simulink model "generic_Truck_And_Trailer"  (R2025a)
settings: Solver=VariableStepAuto  StartTime=0.0  StopTime=350  FixedStep=0.01  MaxStep=0.001  RelTol=1e-3  EnableMultiTasking=on
libraries: TruckMaker4SL x250, simulink x1
(part 3 of 11)

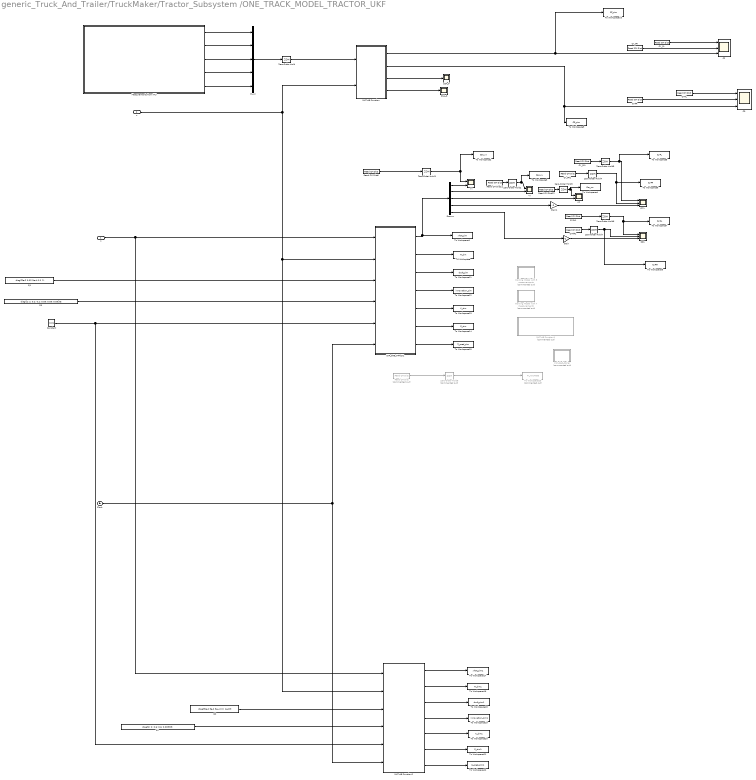
== system generic_Truck_And_Trailer/TruckMaker/Tractor_Subsystem /ONE_TRACK_MODEL_TRACTOR_UKF ==
  z : Inport
  u : Inport  Port=2
  "CF " : Scope  NumInputPorts=3
      settings: ActiveDisplayYMinimum=-12.263034323337607  ActiveDisplayYMaximum=-4.9489164501428942  DataLoggingVariableName=ScopeData23
  CF 1 : Scope  NumInputPorts=3
      settings: ActiveDisplayYMinimum=-10.797860186662938  ActiveDisplayYMaximum=-3.0037046797887497  DataLoggingVariableName=ScopeData30
  CR : Scope  NumInputPorts=3
      settings: ActiveDisplayYMinimum=-11.701585356235972  ActiveDisplayYMaximum=4.5045535239425494  DataLoggingVariableName=ScopeData24
  CR1 : Scope  NumInputPorts=3
      settings: ActiveDisplayYMinimum=-13.474282112558932  ActiveDisplayYMaximum=-8.0648262356989679  DataLoggingVariableName=ScopeData31
  CYRL : TruckMaker4SL/Read CM Dict  xname=CyRL  xsync=off  xstime=Continuous
      settings: SourceProductName=TruckMaker4SL
  CYRL1 : TruckMaker4SL/Read CM Dict  xname=CyRL  xsync=off  xstime=Continuous
      settings: SourceProductName=TruckMaker4SL
  CYRR : TruckMaker4SL/Read CM Dict  xname=CyRR  xsync=off  xstime=Continuous
      settings: SourceProductName=TruckMaker4SL
  CYRR1 : TruckMaker4SL/Read CM Dict  xname=CyRR  xsync=off  xstime=Continuous
      settings: SourceProductName=TruckMaker4SL
  CY_FL : TruckMaker4SL/Read CM Dict  xname=CyFL  xsync=off  xstime=Continuous
      settings: SourceProductName=TruckMaker4SL
  CY_FL1 : TruckMaker4SL/Read CM Dict  xname=CyFL  xsync=off  xstime=Continuous
      settings: SourceProductName=TruckMaker4SL
  CY_FR : TruckMaker4SL/Read CM Dict  xname=CyFR  xsync=off  xstime=Continuous
      settings: SourceProductName=TruckMaker4SL
  CY_FR1 : TruckMaker4SL/Read CM Dict  xname=CyFR  xsync=off  xstime=Continuous
      settings: SourceProductName=TruckMaker4SL
  Clock : Clock
  Constant : Constant  Value=0.01
  Demux : Demux  Outputs=5
  Gain : Gain  Gain=-1
  Gain1 : Gain  Gain=-1
  "Included_trailer " : MATLAB Function  Commented=on  TreatAsAtomicUnit=on
  MATLAB Function : MATLAB Function  TreatAsAtomicUnit=on
  MATLAB Function1 : MATLAB Function  Commented=on  TreatAsAtomicUnit=on
  MATLAB Function2 : MATLAB Function  TreatAsAtomicUnit=on  SystemSampleTime=0.01
  Measurements from IMU : Subsystem  Description=Measurements from IMU Mounted in Vhcl position (3.6; 0.0;1.0)
  Mux2 : Mux  Inputs=5
  Q1 : Constant  Value="diag([2e-2 0.02 3e-4 0 0  ]);"
  Q2 : Constant  Value="diag([5e-2 5e-2 3e-4 0 0  1e-3]);"
  R1 : Constant  Value=diag([2; 2; 0.6; 0.6; 0.005])/3;
  R3 : Constant  Value=diag([2; 2; 0.2; 0.2; 0.05; 0.05; 0.05])/3;
  Read CM Dict : TruckMaker4SL/Read CM Dict  Commented=on  xname=Tr.YawVel  xsync=off  xstime=Continuous
      settings: SourceProductName=TruckMaker4SL
  Read CM Dict11 : TruckMaker4SL/Read CM Dict  xname=Car.vy  xsync=off  xstime=Continuous
      settings: SourceProductName=TruckMaker4SL
  Read CM Dict12 : TruckMaker4SL/Read CM Dict  xname=Car.YawRate  xsync=off  xstime=Continuous
      settings: SourceProductName=TruckMaker4SL
  Read CM Dict6 : TruckMaker4SL/Read CM Dict  xname=Car.vx  xsync=off  xstime=Continuous
      settings: SourceProductName=TruckMaker4SL
  SSA_F : Scope
      settings: ActiveDisplayYMinimum=-0.046315426334515186  ActiveDisplayYMaximum=0.00321973029301955  DataLoggingVariableName=ScopeData25
  SSA_R : Scope
      settings: ActiveDisplayYMinimum=19.809904868748255  ActiveDisplayYMaximum=19.861105266179973  DataLoggingVariableName=ScopeData26
  To Workspace : ToWorkspace  VariableName=P_sim  SaveFormat=Timeseries  SampleTime=-1
  To Workspace1 : ToWorkspace  VariableName=xhat_sim  SaveFormat=Timeseries  SampleTime=-1
  To Workspace10 : ToWorkspace  VariableName=CF_sim  SaveFormat=Timeseries  SampleTime=-1
  To Workspace11 : ToWorkspace  VariableName=dxdt_sim  SaveFormat=Timeseries  SampleTime=-1
  To Workspace12 : ToWorkspace  VariableName=innovation_sim  SaveFormat=Timeseries  SampleTime=-1
  To Workspace13 : ToWorkspace  VariableName=K_sim  SaveFormat=Timeseries  SampleTime=-1
  To Workspace14 : ToWorkspace  VariableName=S_sim  SaveFormat=Timeseries  SampleTime=-1
  To Workspace15 : ToWorkspace  VariableName=Z_pred_sim  SaveFormat=Timeseries  SampleTime=-1
  To Workspace16 : ToWorkspace  VariableName=P_sim1  SaveFormat=Timeseries  SampleTime=-1
  To Workspace17 : ToWorkspace  VariableName=xhat_sim1  SaveFormat=Timeseries  SampleTime=-1
  To Workspace18 : ToWorkspace  VariableName=dxdt_sim1  SaveFormat=Timeseries  SampleTime=-1
  To Workspace19 : ToWorkspace  VariableName=innovation_sim1  SaveFormat=Timeseries  SampleTime=-1
  To Workspace2 : ToWorkspace  VariableName=Car_vx  SaveFormat=Timeseries  SampleTime=-1
  To Workspace20 : ToWorkspace  VariableName=K_sim1  SaveFormat=Timeseries  SampleTime=-1
  To Workspace21 : ToWorkspace  VariableName=S_sim1  SaveFormat=Timeseries  SampleTime=-1
  To Workspace22 : ToWorkspace  VariableName=Z_pred_sim1  SaveFormat=Timeseries  SampleTime=-1
  To Workspace23 : ToWorkspace  Commented=on  VariableName=Tr_YawRate  SaveFormat=Timeseries  SampleTime=-1
  To Workspace3 : ToWorkspace  VariableName=Car_vy  SaveFormat=Timeseries  SampleTime=-1
  To Workspace4 : ToWorkspace  VariableName=Car_wz  SaveFormat=Timeseries  SampleTime=-1
  To Workspace5 : ToWorkspace  VariableName=CyFL  SaveFormat=Timeseries  SampleTime=-1
  To Workspace6 : ToWorkspace  VariableName=CyFR  SaveFormat=Timeseries  SampleTime=-1
  To Workspace7 : ToWorkspace  VariableName=CyRL  SaveFormat=Timeseries  SampleTime=-1
  To Workspace8 : ToWorkspace  VariableName=CyRR  SaveFormat=Timeseries  SampleTime=-1
  To Workspace9 : ToWorkspace  VariableName=CR_sim  SaveFormat=Timeseries  SampleTime=-1
  UKF_ONE_TRACK1 : MATLAB Function  TreatAsAtomicUnit=on  SystemSampleTime=0.01
  "Working Model with 5 measurements " : MATLAB Function  Commented=on  TreatAsAtomicUnit=on
  Working Model with 7 measurements : MATLAB Function  Commented=on  TreatAsAtomicUnit=on
  Zero-Order Hold{,1..7} (8 alike) : ZeroOrderHold  SampleTime=0.01
  Zero-Order Hold8 : ZeroOrderHold  Commented=on  SampleTime=0.01
  vx : Scope  NumInputPorts=2
      settings: ActiveDisplayYMinimum=15.532965030483135  ActiveDisplayYMaximum=19.510688761225374  DataLoggingVariableName=ScopeData34
  vy : Scope  NumInputPorts=2
      settings: ActiveDisplayYMinimum=-0.016234882238860611  ActiveDisplayYMaximum=0.084455127817541567  DataLoggingVariableName=ScopeData35
  wz : Scope  NumInputPorts=2
      settings: ActiveDisplayYMinimum=-0.21237399330212148  ActiveDisplayYMaximum=0.50990512712526215  DataLoggingVariableName=ScopeData36
  wires:
  Zero-Order Hold8/1 -> To Workspace23/1
  Read CM Dict/1 -> Zero-Order Hold8/1
  Zero-Order Hold7/1 -> CR1/2, To Workspace8/1
  Zero-Order Hold6/1 -> CR1/1, To Workspace7/1
  Zero-Order Hold5/1 -> CF 1/1, To Workspace5/1
  Zero-Order Hold4/1 -> CF 1/2, To Workspace6/1
  Zero-Order Hold3/1 -> wz/1, To Workspace4/1
  Zero-Order Hold2/1 -> vy/1, To Workspace3/1
  Zero-Order Hold1/1 -> vx/1, To Workspace2/1
  Zero-Order Hold/1 -> MATLAB Function/1(z)
  Q2/1 -> MATLAB Function2/3(Q)
  R1/1 -> MATLAB Function2/4(R)
  MATLAB Function2/2(P) -> To Workspace16/1
  MATLAB Function2/1(xhat) -> To Workspace17/1  "State_estimates"
  MATLAB Function2/3(dxdt) -> To Workspace18/1
  MATLAB Function2/4(innovation) -> To Workspace19/1
  MATLAB Function2/5(K_out) -> To Workspace20/1
  MATLAB Function2/6(S_out) -> To Workspace21/1
  MATLAB Function2/7(z_pred_out) -> To Workspace22/1
  Clock/1 -> MATLAB Function2/6(data), UKF_ONE_TRACK1/6(data)
  Measurements from IMU/5(wz) -> Mux2/5
  Measurements from IMU/2(acc_y) -> Mux2/2
  Mux2/1 -> Zero-Order Hold/1
  Measurements from IMU/3(vel_x) -> Mux2/3
  Measurements from IMU/4(vel_y) -> Mux2/4
  Measurements from IMU/1(acc_x) -> Mux2/1
  z/1 -> UKF_ONE_TRACK1/1(z), MATLAB Function2/1(z)
  UKF_ONE_TRACK1/7(z_pred_out) -> To Workspace15/1
  UKF_ONE_TRACK1/6(S_out) -> To Workspace14/1
  UKF_ONE_TRACK1/5(K_out) -> To Workspace13/1
  UKF_ONE_TRACK1/4(innovation) -> To Workspace12/1
  u/1 -> UKF_ONE_TRACK1/2(u), MATLAB Function2/2(u), MATLAB Function/2(u)
  Q1/1 -> UKF_ONE_TRACK1/3(Q)
  UKF_ONE_TRACK1/3(dxdt) -> To Workspace11/1
  Gain1/1 -> CF 1/3  "Est_CF"
  Demux/4 -> Gain1/1  "Cmptd_Cf"
  MATLAB Function/3(alpha_f) -> SSA_F/1
  CY_FR/1 -> "CF "/2  "CyFR"
  Demux/3 -> wz/2  "est_wz"
  CY_FL/1 -> "CF "/1  "CyFL"
  Demux/5 -> Gain/1  "cmptd_R"
  Read CM Dict11/1 -> Zero-Order Hold2/1
  CY_FL1/1 -> Zero-Order Hold5/1  "CyFL"
  MATLAB Function/2(Cr) -> CR/3, To Workspace9/1  "cmptd_R"
  Demux/2 -> vy/2  "est_vy"
  CYRR/1 -> CR/2  "CyRR"
  CYRR1/1 -> Zero-Order Hold7/1  "CyRR"
  MATLAB Function/4(alpha_r) -> SSA_R/1
  Read CM Dict12/1 -> Zero-Order Hold3/1
  Constant/1 -> UKF_ONE_TRACK1/5(Ts), MATLAB Function2/5(Ts)
  CYRL/1 -> CR/1  "CyRL"
  Gain/1 -> CR1/3  "est_CR"
  CYRL1/1 -> Zero-Order Hold6/1  "CyRL"
  R3/1 -> UKF_ONE_TRACK1/4(R)
  UKF_ONE_TRACK1/1(xhat) -> To Workspace1/1, Demux/1  "State_estimates"
  UKF_ONE_TRACK1/2(P) -> To Workspace/1
  Demux/1 -> vx/2  "est_vx"
  CY_FR1/1 -> Zero-Order Hold4/1  "CyFR"
  Read CM Dict6/1 -> Zero-Order Hold1/1
  MATLAB Function/1(Cf) -> "CF "/3, To Workspace10/1  "Cmptd_Cf"

== system generic_Truck_And_Trailer/TruckMaker/Tractor_Subsystem /Subsystem ==
  Ackerman Angle : Subsystem  Commented=on
  Average Steering Angle : Subsystem
  Trq_RL : TruckMaker4SL/Read CM Dict  xname=Vhcl.RL.Trq_Drive  xsync=off  xstime=Continuous
      settings: SourceProductName=TruckMaker4SL
  Trq_RR : TruckMaker4SL/Read CM Dict  xname=Vhcl.RR.Trq_Drive  xsync=off  xstime=Continuous
      settings: SourceProductName=TruckMaker4SL
  "Average_steering " : Outport
  Trq_T2W_RL : Outport  Port=2
  Trq_T2W_RR : Outport  Port=3
  wires:
  Average Steering Angle/1("Average_steering ") -> "Average_steering "/1
  Trq_RR/1 -> Trq_T2W_RR/1
  Trq_RL/1 -> Trq_T2W_RL/1

== system generic_Truck_And_Trailer/TruckMaker/Tractor_Subsystem /Subsystem_Noisey Measurements ==
  Acc_x : TruckMaker4SL/Read CM Dict  xname=Vhcl.RL.rotv  xsync=off  xstime=Continuous
      settings: SourceProductName=TruckMaker4SL
  Acc_x1 : TruckMaker4SL/Read CM Dict  xname=Vhcl.RR.rotv  xsync=off  xstime=Continuous
      settings: SourceProductName=TruckMaker4SL
  Demux : Demux  Outputs=2
  Demux1 : Demux  Outputs=2
  Demux2 : Demux  Outputs=2
  Demux3 : Demux  Outputs=1
  MATLAB Function : MATLAB Function  TreatAsAtomicUnit=on
  MATLAB Function1 : MATLAB Function  TreatAsAtomicUnit=on
  MATLAB Function2 : MATLAB Function  TreatAsAtomicUnit=on
  MATLAB Function3 : MATLAB Function  TreatAsAtomicUnit=on
  Measurements from IMU : Subsystem  Description=Measurements from IMU Mounted in Vhcl position (3.6; 0.0;1.0)
  Mux : Mux  Inputs=3
  Mux1 : Mux  Inputs=3
  Mux2 : Mux
  Mux3 : Mux  Inputs=3
  Mux5 : Mux  Inputs=2
  Scope : Scope
      settings: ActiveDisplayYMinimum=-5.6580655588196418  ActiveDisplayYMaximum=20.488387754127984  DataLoggingVariableName=ScopeData37
  Out1 : Outport
  wires:
  MATLAB Function/1(gyro_meas) -> Demux2/1
  MATLAB Function2/1(vel_meas) -> Demux1/1
  MATLAB Function1/1(acc_meas) -> Demux/1
  Demux2/2 -> Mux2/3
  Demux1/1 -> Mux2/2
  Demux/1 -> Mux2/1
  Measurements from IMU/9(wz) -> Mux/3
  Measurements from IMU/8(wy) -> Mux/2
  Measurements from IMU/7(wx) -> Mux/1
  Mux/1 -> MATLAB Function/1(gyro_true)
  Measurements from IMU/6(vel_z) -> Mux1/3
  Measurements from IMU/5(vel_y) -> Mux1/2
  Measurements from IMU/4(vel_x) -> Mux1/1
  Mux3/1 -> MATLAB Function1/1(acc_true)
  Measurements from IMU/1(acc_x) -> Mux3/1
  Measurements from IMU/2(acc_y) -> Mux3/2
  Measurements from IMU/3(acc_z) -> Mux3/3
  Mux2/1 -> Out1/1, Scope/1
  Mux1/1 -> MATLAB Function2/1(truth)
  Acc_x/1 -> Mux5/1
  Acc_x1/1 -> Mux5/2
  Mux5/1 -> MATLAB Function3/1(truth)
  Demux3/1 -> Mux2/4
  MATLAB Function3/1(vel_meas) -> Demux3/1

== system generic_Truck_And_Trailer/TruckMaker/Tractor_Subsystem /Subsystem_Noisey Measurements _NAN ==
  Acc_x : TruckMaker4SL/Read CM Dict  xname=Vhcl.RL.rotv  xsync=off  xstime=Continuous
      settings: SourceProductName=TruckMaker4SL
  Acc_x1 : TruckMaker4SL/Read CM Dict  xname=Vhcl.RR.rotv  xsync=off  xstime=Continuous
      settings: SourceProductName=TruckMaker4SL
  Demux : Demux  Outputs=2
  Demux1 : Demux  Outputs=2
  Demux2 : Demux  Outputs=2
  Demux3 : Demux  Outputs=1
  MATLAB Function : MATLAB Function  TreatAsAtomicUnit=on
  MATLAB Function1 : MATLAB Function  TreatAsAtomicUnit=on
  MATLAB Function2 : MATLAB Function  TreatAsAtomicUnit=on
  MATLAB Function3 : MATLAB Function  TreatAsAtomicUnit=on
  Manual Switch : ManualSwitch  CurrentSetting=0
  Measurements from IMU : Subsystem  Description=Measurements from IMU Mounted in Vhcl position (3.6; 0.0;1.0)
  Mux : Mux  Inputs=3
  Mux1 : Mux  Inputs=3
  Mux2 : Mux
  Mux3 : Mux  Inputs=3
  Mux4 : Mux  Inputs=2
  Mux5 : Mux  Inputs=2
  NaN : Constant  Value=NaN  OutDataTypeStr=Inherit: Inherit via back propagation
  Scope : Scope
      settings: ActiveDisplayYMinimum=-12.833093805155979  ActiveDisplayYMaximum=56.830382589328167  DataLoggingVariableName=ScopeData37
  Out1 : Outport
  wires:
  Manual Switch/1 -> Mux2/2
  Demux1/1 -> Manual Switch/1
  Mux4/1 -> Manual Switch/2
  NaN/1 -> Mux4/2, Mux4/1
  Mux1/1 -> MATLAB Function2/1(truth)
  Mux2/1 -> Out1/1, Scope/1
  Measurements from IMU/3(acc_z) -> Mux3/3
  Measurements from IMU/2(acc_y) -> Mux3/2
  Measurements from IMU/1(acc_x) -> Mux3/1
  Mux3/1 -> MATLAB Function1/1(acc_true)
  Measurements from IMU/4(vel_x) -> Mux1/1
  Measurements from IMU/5(vel_y) -> Mux1/2
  Measurements from IMU/6(vel_z) -> Mux1/3
  Mux/1 -> MATLAB Function/1(gyro_true)
  Measurements from IMU/7(wx) -> Mux/1
  Measurements from IMU/8(wy) -> Mux/2
  Measurements from IMU/9(wz) -> Mux/3
  Demux/1 -> Mux2/1
  Demux2/2 -> Mux2/3
  MATLAB Function1/1(acc_meas) -> Demux/1
  MATLAB Function2/1(vel_meas) -> Demux1/1
  MATLAB Function/1(gyro_meas) -> Demux2/1
  Acc_x/1 -> Mux5/1
  Acc_x1/1 -> Mux5/2
  Mux5/1 -> MATLAB Function3/1(truth)
  Demux3/1 -> Mux2/4
  MATLAB Function3/1(vel_meas) -> Demux3/1

== system generic_Truck_And_Trailer/TruckMaker/VehicleControl/CreateBus Vhcl.Misc ==
  In1 : Inport
  Bus Creator5 : BusCreator  Inputs=11
  Demux5 : Demux  Outputs=11
      settings: DisplayOption=none
  Out1 : Outport  VectorParamsAs1DForOutWhenUnconnected=off
  wires:
  Demux5/11 -> Bus Creator5/11  "Vhcl Wind_vel_0 z"
  Demux5/10 -> Bus Creator5/10  "Vhcl Wind_vel_0 y"
  Demux5/9 -> Bus Creator5/9  "Vhcl Wind_vel_0 x"
  Demux5/8 -> Bus Creator5/8  "Vhcl DL2BdyEng y"
  Demux5/7 -> Bus Creator5/7  "Vhcl DL2BdyEng x"
  Demux5/6 -> Bus Creator5/6  "Vhcl TrqDL2Bdy1B z"
  Demux5/5 -> Bus Creator5/5  "Vhcl TrqDL2Bdy1B y"
  Demux5/4 -> Bus Creator5/4  "Vhcl TrqDL2Bdy1B x"
  Demux5/3 -> Bus Creator5/3  "Vhcl Trq_DL2Bdy1 z"
  In1/1 -> Demux5/1
  Bus Creator5/1 -> Out1/1
  Demux5/2 -> Bus Creator5/2  "Vhcl Trq_DL2Bdy1 y"
  Demux5/1 -> Bus Creator5/1  "Vhcl Trq_DL2Bdy1 x"

== system generic_Truck_And_Trailer/TruckMaker/VehicleControl/CreateBus Vhcl.Wheel.In ==
  In1 : Inport
  Bus Creator1 : BusCreator  Inputs=36
  Demux1 : Demux  Outputs=36
      settings: DisplayOption=none
  Out1 : Outport  VectorParamsAs1DForOutWhenUnconnected=off
  wires:
  Demux1/36 -> Bus Creator1/36  "Vhcl Wheel RR4 rotv"
  Demux1/35 -> Bus Creator1/35  "Vhcl Wheel RR4 Trq_DL2WC"
  Demux1/34 -> Bus Creator1/34  "Vhcl Wheel RR4 Trq_B2WC"
  Demux1/33 -> Bus Creator1/33  "Vhcl Wheel RL4 rotv"
  Demux1/32 -> Bus Creator1/32  "Vhcl Wheel RL4 Trq_DL2WC"
  Demux1/31 -> Bus Creator1/31  "Vhcl Wheel RL4 Trq_B2WC"
  Demux1/30 -> Bus Creator1/30  "Vhcl Wheel RR3 rotv"
  Demux1/29 -> Bus Creator1/29  "Vhcl Wheel RR3 Trq_DL2WC"
  Demux1/28 -> Bus Creator1/28  "Vhcl Wheel RR3 Trq_B2WC"
  Demux1/27 -> Bus Creator1/27  "Vhcl Wheel RL3 rotv"
  Demux1/26 -> Bus Creator1/26  "Vhcl Wheel RL3 Trq_DL2WC"
  Demux1/25 -> Bus Creator1/25  "Vhcl Wheel RL3 Trq_B2WC"
  Demux1/12 -> Bus Creator1/12  "Vhcl Wheel RR rotv"
  Demux1/11 -> Bus Creator1/11  "Vhcl Wheel RR Trq_DL2WC"
  Demux1/10 -> Bus Creator1/10  "Vhcl Wheel RR Trq_B2WC"
  Demux1/9 -> Bus Creator1/9  "Vhcl Wheel RL rotv"
  Demux1/8 -> Bus Creator1/8  "Vhcl Wheel RL Trq_DL2WC"
  Demux1/7 -> Bus Creator1/7  "Vhcl Wheel RL Trq_B2WC"
  Demux1/6 -> Bus Creator1/6  "Vhcl Wheel FR rotv"
  Demux1/5 -> Bus Creator1/5  "Vhcl Wheel FR Trq_DL2WC"
  Demux1/4 -> Bus Creator1/4  "Vhcl Wheel FR Trq_B2WC"
  Demux1/3 -> Bus Creator1/3  "Vhcl Wheel FL rotv"
  Demux1/2 -> Bus Creator1/2  "Vhcl Wheel FL Trq_DL2WC"
  Demux1/1 -> Bus Creator1/1  "Vhcl Wheel FL Trq_B2WC"
  Bus Creator1/1 -> Out1/1
  In1/1 -> Demux1/1
  Demux1/24 -> Bus Creator1/24  "Vhcl Wheel FR2 rotv"
  Demux1/23 -> Bus Creator1/23  "Vhcl Wheel FR2 Trq_DL2WC"
  Demux1/22 -> Bus Creator1/22  "Vhcl Wheel FR2 Trq_B2WC"
  Demux1/21 -> Bus Creator1/21  "Vhcl Wheel FL2 rotv"
  Demux1/20 -> Bus Creator1/20  "Vhcl Wheel FL2 Trq_DL2WC"
  Demux1/19 -> Bus Creator1/19  "Vhcl Wheel FL2 Trq_B2WC"
  Demux1/18 -> Bus Creator1/18  "Vhcl Wheel RR2 rotv"
  Demux1/17 -> Bus Creator1/17  "Vhcl Wheel RR2 Trq_DL2WC"
  Demux1/16 -> Bus Creator1/16  "Vhcl Wheel RR2 Trq_B2WC"
  Demux1/15 -> Bus Creator1/15  "Vhcl Wheel RL2 rotv"
  Demux1/14 -> Bus Creator1/14  "Vhcl Wheel RL2 Trq_DL2WC"
  Demux1/13 -> Bus Creator1/13  "Vhcl Wheel RL2 Trq_B2WC"

== system generic_Truck_And_Trailer/TruckMaker/VehicleControl/CreateBus VhclCtrl ==
  In : Inport
  BusCreator : BusCreator  Inputs=29
  Demux : Demux  Outputs=29
      settings: DisplayOption=none
  Out : Outport  VectorParamsAs1DForOutWhenUnconnected=off
  wires:
  Demux/29 -> BusCreator/29  "VhclCtrl Lights Reverse"
  Demux/28 -> BusCreator/28  "VhclCtrl Lights Brake"
  Demux/27 -> BusCreator/27  "VhclCtrl Lights FogRear"
  Demux/26 -> BusCreator/26  "VhclCtrl Lights FogFrontR"
  Demux/25 -> BusCreator/25  "VhclCtrl Lights FogFrontL"
  Demux/24 -> BusCreator/24  "VhclCtrl Lights IndR"
  Demux/23 -> BusCreator/23  "VhclCtrl Lights IndL"
  Demux/22 -> BusCreator/22  "VhclCtrl Lights ParkR"
  Demux/21 -> BusCreator/21  "VhclCtrl Lights ParkL"
  Demux/20 -> BusCreator/20  "VhclCtrl Lights Daytime"
  Demux/19 -> BusCreator/19  "VhclCtrl Lights HighBeam"
  Demux/18 -> BusCreator/18  "VhclCtrl Lights LowBeam"
  Demux/17 -> BusCreator/17  "VhclCtrl Steering Trq"
  Demux/16 -> BusCreator/16  "VhclCtrl Steering AngAcc"
  Demux/15 -> BusCreator/15  "VhclCtrl Steering AngVel"
  Demux/14 -> BusCreator/14  "VhclCtrl Steering Ang"
  Demux/13 -> BusCreator/13  "VhclCtrl Gas"
  Demux/12 -> BusCreator/12  "VhclCtrl Clutch"
  Demux/11 -> BusCreator/11  "VhclCtrl BrakePark"
  Demux/10 -> BusCreator/10  "VhclCtrl Brake"
  Demux/9 -> BusCreator/9  "VhclCtrl SelectorCtrl"
  Demux/8 -> BusCreator/8  "VhclCtrl GearNo"
  Demux/7 -> BusCreator/7  "VhclCtrl UserSignal4"
  Demux/6 -> BusCreator/6  "VhclCtrl UserSignal3"
  Demux/5 -> BusCreator/5  "VhclCtrl UserSignal2"
  Demux/4 -> BusCreator/4  "VhclCtrl UserSignal1"
  Demux/3 -> BusCreator/3  "VhclCtrl UserSignal0"
  Demux/2 -> BusCreator/2  "VhclCtrl Key"
  Demux/1 -> BusCreator/1  "VhclCtrl SST"
  BusCreator/1 -> Out/1
  In/1 -> Demux/1

== system generic_Truck_And_Trailer/TruckMaker/VehicleControl/CreateBus VhclCtrl.PT ==
  In1 : Inport
  BusCreator1 : BusCreator  Inputs=12
  Demux1 : Demux  Outputs=12
      settings: DisplayOption=none
  Out1 : Outport  VectorParamsAs1DForOutWhenUnconnected=off
  wires:
  BusCreator1/1 -> Out1/1
  In1/1 -> Demux1/1
  Demux1/1 -> BusCreator1/1  "VhclCtrl SST"
  Demux1/2 -> BusCreator1/2  "VhclCtrl Key"
  Demux1/3 -> BusCreator1/3  "VhclCtrl UserSignal0"
  Demux1/4 -> BusCreator1/4  "VhclCtrl UserSignal1"
  Demux1/5 -> BusCreator1/5  "VhclCtrl UserSignal2"
  Demux1/6 -> BusCreator1/6  "VhclCtrl UserSignal3"
  Demux1/7 -> BusCreator1/7  "VhclCtrl UserSignal4"
  Demux1/8 -> BusCreator1/8  "VhclCtrl GearNo"
  Demux1/9 -> BusCreator1/9  "VhclCtrl SelectorCtrl"
  Demux1/10 -> BusCreator1/10  "VhclCtrl Clutch"
  Demux1/11 -> BusCreator1/11  "VhclCtrl Gas"
  Demux1/12 -> BusCreator1/12  "VhclCtrl Brake"

== system generic_Truck_And_Trailer/TruckMaker/VehicleControl/CreateBus VhclCtrl.Steering ==
  In1 : Inport
  Bus Creator : BusCreator  Inputs=5
  Demux : Demux  Outputs=5
      settings: DisplayOption=none
  Out1 : Outport  VectorParamsAs1DForOutWhenUnconnected=off
  wires:
  In1/1 -> Demux/1
  Bus Creator/1 -> Out1/1
  Demux/1 -> Bus Creator/1  "VhclCtrl Steering Ang"
  Demux/5 -> Bus Creator/5  "VhclCtrl Steering ByTrq"
  Demux/3 -> Bus Creator/3  "VhclCtrl Steering AngAcc"
  Demux/2 -> Bus Creator/2  "VhclCtrl Steering AngVel"
  Demux/4 -> Bus Creator/4  "VhclCtrl Steering Trq"

== system generic_Truck_And_Trailer/TruckMaker/IPG Vehicle/Brake/CreateBus Vhcl.Wheel.PT ==
  In : Inport
  BusCreator : BusCreator  Inputs=60
  Demux : Demux  Outputs=60
      settings: DisplayOption=none
  Out : Outport  VectorParamsAs1DForOutWhenUnconnected=off
  wires:
  Demux/60 -> BusCreator/60  "Vhcl Trq_DriveSrc_trg d11"
  Demux/59 -> BusCreator/59  "Vhcl Trq_DriveSrc_trg d10"
  Demux/58 -> BusCreator/58  "Vhcl Trq_DriveSrc_trg d9"
  Demux/57 -> BusCreator/57  "Vhcl Trq_DriveSrc_trg d8"
  Demux/56 -> BusCreator/56  "Vhcl Trq_DriveSrc_trg d7"
  Demux/55 -> BusCreator/55  "Vhcl Trq_DriveSrc_trg d6"
  Demux/54 -> BusCreator/54  "Vhcl Trq_DriveSrc_trg d5"
  Demux/53 -> BusCreator/53  "Vhcl Trq_DriveSrc_trg d4"
  Demux/52 -> BusCreator/52  "Vhcl Trq_DriveSrc_trg d3"
  Demux/51 -> BusCreator/51  "Vhcl Trq_DriveSrc_trg d2"
  Demux/50 -> BusCreator/50  "Vhcl Trq_DriveSrc_trg d1"
  Demux/49 -> BusCreator/49  "Vhcl Trq_DriveSrc_trg d0"
  Demux/48 -> BusCreator/48  "Vhcl Wheel RR4 WhlBearing"
  Demux/47 -> BusCreator/47  "Vhcl Wheel RR4 Trq_T2W"
  Demux/46 -> BusCreator/46  "Vhcl Wheel RR4 Trq_BrakeReg_trg"
  Demux/45 -> BusCreator/45  "Vhcl Wheel RR4 Trq_Brake"
  Demux/44 -> BusCreator/44  "Vhcl Wheel RL4 WhlBearing"
  Demux/43 -> BusCreator/43  "Vhcl Wheel RL4 Trq_T2W"
  Demux/42 -> BusCreator/42  "Vhcl Wheel RL4 Trq_BrakeReg_trg"
  Demux/41 -> BusCreator/41  "Vhcl Wheel RL4 Trq_Brake"
  Demux/40 -> BusCreator/40  "Vhcl Wheel RR3 WhlBearing"
  Demux/39 -> BusCreator/39  "Vhcl Wheel RR3 Trq_T2W"
  Demux/38 -> BusCreator/38  "Vhcl Wheel RR3 Trq_BrakeReg_trg"
  Demux/37 -> BusCreator/37  "Vhcl Wheel RR3 Trq_Brake"
  Demux/36 -> BusCreator/36  "Vhcl Wheel RL3 WhlBearing"
  Demux/35 -> BusCreator/35  "Vhcl Wheel RL3 Trq_T2W"
  Demux/34 -> BusCreator/34  "Vhcl Wheel RL3 Trq_BrakeReg_trg"
  Demux/33 -> BusCreator/33  "Vhcl Wheel RL3 Trq_Brake"
  Demux/32 -> BusCreator/32  "Vhcl Wheel FR2 WhlBearing"
  Demux/31 -> BusCreator/31  "Vhcl Wheel FR2 Trq_T2W"
  Demux/30 -> BusCreator/30  "Vhcl Wheel FR2 Trq_BrakeReg_trg"
  Demux/29 -> BusCreator/29  "Vhcl Wheel FR2 Trq_Brake"
  Demux/28 -> BusCreator/28  "Vhcl Wheel FL2 WhlBearing"
  Demux/27 -> BusCreator/27  "Vhcl Wheel FL2 Trq_T2W"
  Demux/26 -> BusCreator/26  "Vhcl Wheel FL2 Trq_BrakeReg_trg"
  Demux/25 -> BusCreator/25  "Vhcl Wheel FL2 Trq_Brake"
  Demux/24 -> BusCreator/24  "Vhcl Wheel RR2 WhlBearing"
  Demux/23 -> BusCreator/23  "Vhcl Wheel RR2 Trq_T2W"
  Demux/22 -> BusCreator/22  "Vhcl Wheel RR2 Trq_BrakeReg_trg"
  Demux/21 -> BusCreator/21  "Vhcl Wheel RR2 Trq_Brake"
  Demux/20 -> BusCreator/20  "Vhcl Wheel RL2 WhlBearing"
  Demux/19 -> BusCreator/19  "Vhcl Wheel RL2 Trq_T2W"
  Demux/18 -> BusCreator/18  "Vhcl Wheel RL2 Trq_BrakeReg_trg"
  Demux/17 -> BusCreator/17  "Vhcl Wheel RL2 Trq_Brake"
  Demux/16 -> BusCreator/16  "Vhcl Wheel RR WhlBearing"
  Demux/15 -> BusCreator/15  "Vhcl Wheel RR Trq_T2W"
  Demux/14 -> BusCreator/14  "Vhcl Wheel RR Trq_BrakeReg_trg"
  Demux/13 -> BusCreator/13  "Vhcl Wheel RR Trq_Brake"
  Demux/12 -> BusCreator/12  "Vhcl Wheel RL WhlBearing"
  Demux/11 -> BusCreator/11  "Vhcl Wheel RL Trq_T2W"
  Demux/10 -> BusCreator/10  "Vhcl Wheel RL Trq_BrakeReg_trg"
  Demux/9 -> BusCreator/9  "Vhcl Wheel RL Trq_Brake"
  Demux/8 -> BusCreator/8  "Vhcl Wheel FR WhlBearing"
  Demux/7 -> BusCreator/7  "Vhcl Wheel FR Trq_T2W"
  Demux/6 -> BusCreator/6  "Vhcl Wheel FR Trq_BrakeReg_trg"
  Demux/5 -> BusCreator/5  "Vhcl Wheel FR Trq_Brake"
  Demux/4 -> BusCreator/4  "Vhcl Wheel FL WhlBearing"
  Demux/3 -> BusCreator/3  "Vhcl Wheel FL Trq_T2W"
  Demux/2 -> BusCreator/2  "Vhcl Wheel FL Trq_BrakeReg_trg"
  Demux/1 -> BusCreator/1  "Vhcl Wheel FL Trq_Brake"
  BusCreator/1 -> Out/1
  In/1 -> Demux/1

== system generic_Truck_And_Trailer/TruckMaker/IPG Vehicle/CarAndTrailer/CarAndTrailerUpd ==
  Sync_In : Inport
  Vhcl.Steering : Inport  Port=2
  Vhcl.Motion : Inport  Port=3
  Vhcl.PoI : Inport  Port=4
  Vhcl.Wheel.FL : Inport  Port=5
  Vhcl.Wheel.FR : Inport  Port=6
  Vhcl.Wheel.RL : Inport  Port=7
  Vhcl.Wheel.RR : Inport  Port=8
  Vhcl.Wheel.RL2 : Inport  Port=9
  Vhcl.Wheel.RR2 : Inport  Port=10
  Vhcl.Wheel.FL2 : Inport  Port=11
  Vhcl.Wheel.FR2 : Inport  Port=12
  Vhcl.Wheel.RL3 : Inport  Port=13
  Vhcl.Wheel.RR3 : Inport  Port=14
  Vhcl.Wheel.RL4 : Inport  Port=15
  Vhcl.Wheel.RR4 : Inport  Port=16
  Car.Hitch.FrcTrq : Inport  Port=17
  Vhcl.Fr1A : Inport  Port=18
  CarAndTrailerUpd : S-Function  FunctionName=TM_Sfun  Parameters='CarAndTrUpd'  SFunctionDeploymentMode=off  EnableBusSupport=off
  CreateBus Brake.IF.In : Subsystem
  Sync_Out : Outport  VectorParamsAs1DForOutWhenUnconnected=off
  Brake.IF.In : Outport  Port=2  VectorParamsAs1DForOutWhenUnconnected=off
  wires:
  Vhcl.Wheel.RL3/1 -> CarAndTrailerUpd/13
  Vhcl.Wheel.RR3/1 -> CarAndTrailerUpd/14
  Vhcl.Wheel.RL4/1 -> CarAndTrailerUpd/15
  Vhcl.Wheel.RR4/1 -> CarAndTrailerUpd/16
  Vhcl.Fr1A/1 -> CarAndTrailerUpd/18  "user vehicle only"
  Vhcl.Wheel.RL2/1 -> CarAndTrailerUpd/9
  Vhcl.Wheel.RR2/1 -> CarAndTrailerUpd/10
  Vhcl.Wheel.FL2/1 -> CarAndTrailerUpd/11
  Vhcl.Wheel.FR2/1 -> CarAndTrailerUpd/12
  Car.Hitch.FrcTrq/1 -> CarAndTrailerUpd/17
  Vhcl.Wheel.RR/1 -> CarAndTrailerUpd/8
  Vhcl.Wheel.RL/1 -> CarAndTrailerUpd/7
  Vhcl.Wheel.FR/1 -> CarAndTrailerUpd/6
  Vhcl.Wheel.FL/1 -> CarAndTrailerUpd/5
  Vhcl.Steering/1 -> CarAndTrailerUpd/2
  Vhcl.Motion/1 -> CarAndTrailerUpd/3
  Vhcl.PoI/1 -> CarAndTrailerUpd/4
  CarAndTrailerUpd/2 -> CreateBus Brake.IF.In/1(In)
  CreateBus Brake.IF.In/1(Out) -> Brake.IF.In/1
  CarAndTrailerUpd/1 -> Sync_Out/1
  Sync_In/1 -> CarAndTrailerUpd/1

== system generic_Truck_And_Trailer/TruckMaker/IPG Vehicle/CarAndTrailer/Forces ==
  Sync_In : Inport
  lSpring : Inport  Port=2
  vDamp : Inport  Port=3
  lStabi : Inport  Port=4
  lBuf : Inport  Port=5
  tWheelCarrier_z : Inport  Port=6
  Suspension Forces : Subsystem
  Vehicle Forces : Subsystem
  Sync_Out : Outport  VectorParamsAs1DForOutWhenUnconnected=off
  Car.Virtual : Outport  Port=2  VectorParamsAs1DForOutWhenUnconnected=off
  Car.Aero : Outport  Port=3  VectorParamsAs1DForOutWhenUnconnected=off
  Car.Load : Outport  Port=4  VectorParamsAs1DForOutWhenUnconnected=off
  wires:
  Suspension Forces/1(Sync_Out) -> Sync_Out/1
  Vehicle Forces/1(Sync_Out) -> Suspension Forces/1(Sync_In)
  lBuf/1 -> Suspension Forces/5(lBuf)
  lStabi/1 -> Suspension Forces/4(lStabi)
  vDamp/1 -> Suspension Forces/3(vDamp)
  lSpring/1 -> Suspension Forces/2(lSpring)
  Vehicle Forces/4(Car.Load) -> Car.Load/1
  Vehicle Forces/3(Car.Aero) -> Car.Aero/1
  Vehicle Forces/2(Car.Virtual) -> Car.Virtual/1
  Sync_In/1 -> Vehicle Forces/1(Sync_In)
  tWheelCarrier_z/1 -> Suspension Forces/6(tWheelCarrier_z)

== system generic_Truck_And_Trailer/TruckMaker/IPG Vehicle/CarAndTrailer/Kinematics ==
  Sync_In : Inport
  Steer.IF : Inport  Port=2
  Kinematics : S-Function  FunctionName=TM_Sfun  Parameters='Kinematics'  SFunctionDeploymentMode=off  EnableBusSupport=off
  TireFL.In : Terminator
  TireFR.In : Terminator
  TireRL.In : Terminator
  TireRR.In : Terminator
  Sync_Out : Outport  VectorParamsAs1DForOutWhenUnconnected=off
  lSpring : Outport  Port=2  VectorParamsAs1DForOutWhenUnconnected=off
  vDamp : Outport  Port=3  VectorParamsAs1DForOutWhenUnconnected=off
  lStabi : Outport  Port=4  VectorParamsAs1DForOutWhenUnconnected=off
  lBuf : Outport  Port=5  VectorParamsAs1DForOutWhenUnconnected=off
  tWheelCarrier_z : Outport  Port=6  VectorParamsAs1DForOutWhenUnconnected=off
  wires:
  Kinematics/8 -> lStabi/1
  Kinematics/2 -> TireFL.In/1
  Kinematics/3 -> TireFR.In/1
  Kinematics/4 -> TireRL.In/1
  Kinematics/5 -> TireRR.In/1
  Kinematics/6 -> lSpring/1
  Kinematics/7 -> vDamp/1
  Sync_In/1 -> Kinematics/1
  Kinematics/1 -> Sync_Out/1
  Steer.IF/1 -> Kinematics/2
  Kinematics/9 -> lBuf/1
  Kinematics/10 -> tWheelCarrier_z/1

== system generic_Truck_And_Trailer/TruckMaker/IPG Vehicle/CarAndTrailer/Kinetics ==
  Sync_In : Inport
  Car.Virtual : Inport  Port=2
  Car.Aero : Inport  Port=3
  Car.Load : Inport  Port=4
  Bus Creator : BusCreator  Inputs=20
  Bus Creator1 : BusCreator  Inputs=12
  Bus Creator2 : BusCreator  Inputs=6
  Bus Creator3 : BusCreator  Inputs=6
  Bus Creator4 : BusCreator  Inputs=4
  Demux : Demux  Outputs=12
      settings: DisplayOption=none
  Demux1 : Demux  Outputs=6
      settings: DisplayOption=none
  Demux2 : Demux  Outputs=6
      settings: DisplayOption=none
  Demux3 : Demux
      settings: DisplayOption=none
  Demux4 : Demux  Outputs=20
      settings: DisplayOption=none
  Kinetics : S-Function  FunctionName=TM_Sfun  Parameters='Kinetics'  SFunctionDeploymentMode=off  EnableBusSupport=off
  TireFL.Out : Ground
  TireFR.Out : Ground
  TireRL.Out : Ground
  TireRR.Out : Ground
  Sync_Out : Outport  VectorParamsAs1DForOutWhenUnconnected=off
  Trailer.Load : Outport  Port=2  VectorParamsAs1DForOutWhenUnconnected=off
  Car.Hitch : Outport  Port=3  VectorParamsAs1DForOutWhenUnconnected=off
  Car.Fr1 : Outport  Port=4  VectorParamsAs1DForOutWhenUnconnected=off
  Car.Trq_T2W : Outport  Port=5  VectorParamsAs1DForOutWhenUnconnected=off
  WheelCarrier.Misc : Outport  Port=6  VectorParamsAs1DForOutWhenUnconnected=off
  wires:
  Demux4/20 -> Bus Creator/20  "Car Trq_T2WRR4Twin"
  Demux4/19 -> Bus Creator/19  "Car Trq_T2WRR4"
  Demux4/18 -> Bus Creator/18  "Car Trq_T2WRL4Twin"
  Demux4/17 -> Bus Creator/17  "Car Trq_T2WRL4"
  Demux4/16 -> Bus Creator/16  "Car Trq_T2WRR3Twin"
  Demux4/15 -> Bus Creator/15  "Car Trq_T2WRR3"
  Demux4/14 -> Bus Creator/14  "Car Trq_T2WRL3Twin"
  Demux4/13 -> Bus Creator/13  "Car Trq_T2WRL3"
  Demux4/12 -> Bus Creator/12  "Car Trq_T2WFR2"
  Demux4/11 -> Bus Creator/11  "Car Trq_T2WFL2"
  Sync_In/1 -> Kinetics/1
  Kinetics/1 -> Sync_Out/1
  Car.Aero/1 -> Kinetics/3
  Car.Virtual/1 -> Kinetics/2
  Bus Creator1/1 -> Trailer.Load/1
  Demux/1 -> Bus Creator1/1  "Trailer Load_0 mass"
  Demux/2 -> Bus Creator1/2  "Trailer Load_0 tx"
  Demux/3 -> Bus Creator1/3  "Trailer Load_0 ty"
  Demux/4 -> Bus Creator1/4  "Trailer Load_0 tz"
  Kinetics/2 -> Demux/1
  Demux/5 -> Bus Creator1/5  "Trailer Load_1 mass"
  Demux/6 -> Bus Creator1/6  "Trailer Load_1 tx"
  Demux/7 -> Bus Creator1/7  "Trailer Load_1 ty"
  Demux/8 -> Bus Creator1/8  "Trailer Load_1 tz"
  Demux/9 -> Bus Creator1/9  "Trailer Load_2 mass"
  Demux/10 -> Bus Creator1/10  "Trailer Load_2 tx"
  Demux/11 -> Bus Creator1/11  "Trailer Load_2 ty"
  Demux/12 -> Bus Creator1/12  "Trailer Load_2 tz"
  Demux1/1 -> Bus Creator2/1  "Car Hitch tx"
  Demux1/2 -> Bus Creator2/2  "Car Hitch ty"
  Demux1/3 -> Bus Creator2/3  "Car Hitch tz"
  Demux1/4 -> Bus Creator2/4  "Car Hitch vx"
  Demux1/5 -> Bus Creator2/5  "Car Hitch vy"
  Demux1/6 -> Bus Creator2/6  "Car Hitch vz"
  Kinetics/3 -> Demux1/1
  Bus Creator2/1 -> Car.Hitch/1
  Demux2/1 -> Bus Creator3/1  "Car Fr1 rx"
  Demux2/2 -> Bus Creator3/2  "Car Fr1 ry"
  Demux2/3 -> Bus Creator3/3  "Car Fr1 rz"
  Demux2/4 -> Bus Creator3/4  "Car Fr1 rvx"
  Demux2/5 -> Bus Creator3/5  "Car Fr1 rvy"
  Demux2/6 -> Bus Creator3/6  "Car Fr1 rvz"
  Bus Creator3/1 -> Car.Fr1/1
  Kinetics/4 -> Demux2/1
  Car.Load/1 -> Kinetics/4
  Demux3/1 -> Bus Creator4/1  "car Susp FL GenInert2"
  Demux3/2 -> Bus Creator4/2  "car Susp FR GenInert2"
  Demux3/3 -> Bus Creator4/3  "car Susp FL GenFrc2"
  Demux3/4 -> Bus Creator4/4  "car Susp FR GenFrc2"
  Bus Creator4/1 -> WheelCarrier.Misc/1
  Demux4/3 -> Bus Creator/3  "Car Trq_T2WRL"
  Demux4/2 -> Bus Creator/2  "Car Trq_T2WFR"
  Demux4/1 -> Bus Creator/1  "Car Trq_T2WFL"
  TireFL.Out/1 -> Kinetics/5
  TireFR.Out/1 -> Kinetics/6
  TireRL.Out/1 -> Kinetics/7
  TireRR.Out/1 -> Kinetics/8
  Kinetics/6 -> Demux3/1
  Kinetics/5 -> Demux4/1
  Bus Creator/1 -> Car.Trq_T2W/1
  Demux4/9 -> Bus Creator/9  "Car Trq_T2WRR2"
  Demux4/10 -> Bus Creator/10  "Car Trq_T2WRR2Twin"
  Demux4/7 -> Bus Creator/7  "Car Trq_T2WRL2"
  Demux4/8 -> Bus Creator/8  "Car Trq_T2WRL2Twin"
  Demux4/5 -> Bus Creator/5  "Car Trq_T2WRR"
  Demux4/4 -> Bus Creator/4  "Car Trq_T2WRLTwin"
  Demux4/6 -> Bus Creator/6  "Car Trq_T2WRRTwin"

== system generic_Truck_And_Trailer/TruckMaker/IPG Vehicle/CarAndTrailer/Steering ==
  note: When replacing the entire steering system,
      | be sure to disable the IPG steering model by using the steering
      | model 'Model Manager off' in the vehicle GUI.
  Sync_In : Inport
  VhclCtrl.Steering : Inport  Port=2
  Bus Creator1 : BusCreator  Inputs=16
  Bus Creator2 : BusCreator  Inputs=5
  Demux : Demux  Outputs=21
      settings: DisplayOption=none
  Steering : S-Function  FunctionName=TM_Sfun  Parameters='Steering'  SFunctionDeploymentMode=off  EnableBusSupport=off
  Terminator : Terminator
  Sync_Out : Outport  VectorParamsAs1DForOutWhenUnconnected=off
  Steer.IF : Outport  Port=2  VectorParamsAs1DForOutWhenUnconnected=off
  wires:
  Demux/21 -> Bus Creator2/5  "Steering IF R Inert"
  Demux/20 -> Bus Creator2/4  "Steering IF R Frc"
  Demux/19 -> Bus Creator2/3  "Steering IF L Inert"
  Demux/18 -> Bus Creator2/2  "Steering IF L Frc"
  Demux/17 -> Bus Creator2/1  "Steering IF SteerByTrq"
  Demux/16 -> Bus Creator1/16  "Steering IF R iSteer2q"
  Demux/15 -> Bus Creator1/15  "Steering IF R qpp"
  Demux/14 -> Bus Creator1/14  "Steering IF R qp"
  Demux/13 -> Bus Creator1/13  "Steering IF R q"
  Demux/12 -> Bus Creator1/12  "Steering IF L iSteer2q"
  Demux/11 -> Bus Creator1/11  "Steering IF L qpp"
  Demux/10 -> Bus Creator1/10  "Steering IF L qp"
  Demux/9 -> Bus Creator1/9  "Steering IF L q"
  Demux/8 -> Bus Creator1/8  "Steering IF AssistTrqPin"
  Demux/7 -> Bus Creator1/7  "Steering IF AssistTrqCol"
  Demux/6 -> Bus Creator1/6  "Steering IF AssistFrc"
  Demux/5 -> Bus Creator1/5  "Steering IF TrqStatic"
  Demux/4 -> Bus Creator1/4  "Steering IF Trq"
  Demux/3 -> Bus Creator1/3  "Steering IF AngAcc"
  Demux/2 -> Bus Creator1/2  "Steering IF AngVel"
  Demux/1 -> Bus Creator1/1  "Steering IF Ang"
  Bus Creator1/1 -> Steer.IF/1
  Bus Creator2/1 -> Terminator/1  "Steer IF (in)"
  Sync_In/1 -> Steering/1
  Steering/1 -> Sync_Out/1
  VhclCtrl.Steering/1 -> Steering/2
  Steering/2 -> Demux/1

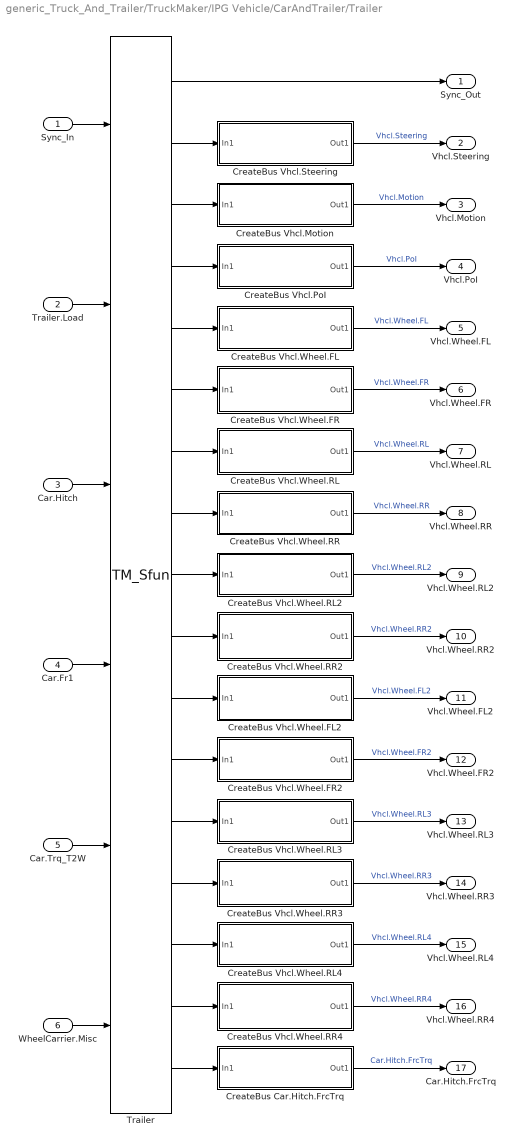
== system generic_Truck_And_Trailer/TruckMaker/IPG Vehicle/CarAndTrailer/Trailer ==
  Sync_In : Inport
  Trailer.Load : Inport  Port=2
  Car.Hitch : Inport  Port=3
  Car.Fr1 : Inport  Port=4
  Car.Trq_T2W : Inport  Port=5
  WheelCarrier.Misc : Inport  Port=6
  CreateBus Car.Hitch.FrcTrq : Subsystem
  CreateBus Vhcl.Motion : Subsystem
  CreateBus Vhcl.PoI : Subsystem
  CreateBus Vhcl.Steering : Subsystem
  CreateBus Vhcl.Wheel.FL : Subsystem
  CreateBus Vhcl.Wheel.FL2 : Subsystem
  CreateBus Vhcl.Wheel.FR : Subsystem
  CreateBus Vhcl.Wheel.FR2 : Subsystem
  CreateBus Vhcl.Wheel.RL : Subsystem
  CreateBus Vhcl.Wheel.RL2 : Subsystem
  CreateBus Vhcl.Wheel.RL3 : Subsystem
  CreateBus Vhcl.Wheel.RL4 : Subsystem
  CreateBus Vhcl.Wheel.RR : Subsystem
  CreateBus Vhcl.Wheel.RR2 : Subsystem
  CreateBus Vhcl.Wheel.RR3 : Subsystem
  CreateBus Vhcl.Wheel.RR4 : Subsystem
  Trailer : S-Function  FunctionName=TM_Sfun  Parameters='Trailer'  SFunctionDeploymentMode=off  EnableBusSupport=off
  Sync_Out : Outport  VectorParamsAs1DForOutWhenUnconnected=off
  Vhcl.Steering : Outport  Port=2  VectorParamsAs1DForOutWhenUnconnected=off
  Vhcl.Motion : Outport  Port=3  VectorParamsAs1DForOutWhenUnconnected=off
  Vhcl.PoI : Outport  Port=4  VectorParamsAs1DForOutWhenUnconnected=off
  Vhcl.Wheel.FL : Outport  Port=5  VectorParamsAs1DForOutWhenUnconnected=off
  Vhcl.Wheel.FR : Outport  Port=6  VectorParamsAs1DForOutWhenUnconnected=off
  Vhcl.Wheel.RL : Outport  Port=7  VectorParamsAs1DForOutWhenUnconnected=off
  Vhcl.Wheel.RR : Outport  Port=8  VectorParamsAs1DForOutWhenUnconnected=off
  Vhcl.Wheel.RL2 : Outport  Port=9  VectorParamsAs1DForOutWhenUnconnected=off
  Vhcl.Wheel.RR2 : Outport  Port=10  VectorParamsAs1DForOutWhenUnconnected=off
  Vhcl.Wheel.FL2 : Outport  Port=11  VectorParamsAs1DForOutWhenUnconnected=off
  Vhcl.Wheel.FR2 : Outport  Port=12  VectorParamsAs1DForOutWhenUnconnected=off
  Vhcl.Wheel.RL3 : Outport  Port=13  VectorParamsAs1DForOutWhenUnconnected=off
  Vhcl.Wheel.RR3 : Outport  Port=14  VectorParamsAs1DForOutWhenUnconnected=off
  Vhcl.Wheel.RL4 : Outport  Port=15  VectorParamsAs1DForOutWhenUnconnected=off
  Vhcl.Wheel.RR4 : Outport  Port=16  VectorParamsAs1DForOutWhenUnconnected=off
  Car.Hitch.FrcTrq : Outport  Port=17  VectorParamsAs1DForOutWhenUnconnected=off
  wires:
  Trailer/16 -> CreateBus Vhcl.Wheel.RR4/1(In1)
  Trailer/15 -> CreateBus Vhcl.Wheel.RL4/1(In1)
  Trailer/14 -> CreateBus Vhcl.Wheel.RR3/1(In1)
  Trailer/13 -> CreateBus Vhcl.Wheel.RL3/1(In1)
  CreateBus Vhcl.Wheel.RL4/1(Out1) -> Vhcl.Wheel.RL4/1  "Vhcl.Wheel.RL4"
  CreateBus Vhcl.Wheel.RR4/1(Out1) -> Vhcl.Wheel.RR4/1  "Vhcl.Wheel.RR4"
  CreateBus Vhcl.Wheel.RR3/1(Out1) -> Vhcl.Wheel.RR3/1  "Vhcl.Wheel.RR3"
  CreateBus Vhcl.Wheel.RL3/1(Out1) -> Vhcl.Wheel.RL3/1  "Vhcl.Wheel.RL3"
  CreateBus Vhcl.Wheel.RL2/1(Out1) -> Vhcl.Wheel.RL2/1  "Vhcl.Wheel.RL2"
  CreateBus Vhcl.Wheel.RR2/1(Out1) -> Vhcl.Wheel.RR2/1  "Vhcl.Wheel.RR2"
  CreateBus Vhcl.Wheel.FL2/1(Out1) -> Vhcl.Wheel.FL2/1  "Vhcl.Wheel.FL2"
  CreateBus Vhcl.Wheel.FR2/1(Out1) -> Vhcl.Wheel.FR2/1  "Vhcl.Wheel.FR2"
  Trailer/12 -> CreateBus Vhcl.Wheel.FR2/1(In1)
  Trailer/11 -> CreateBus Vhcl.Wheel.FL2/1(In1)
  Trailer/10 -> CreateBus Vhcl.Wheel.RR2/1(In1)
  Trailer/9 -> CreateBus Vhcl.Wheel.RL2/1(In1)
  CreateBus Vhcl.Wheel.FL/1(Out1) -> Vhcl.Wheel.FL/1  "Vhcl.Wheel.FL"
  CreateBus Vhcl.Wheel.FR/1(Out1) -> Vhcl.Wheel.FR/1  "Vhcl.Wheel.FR"
  CreateBus Vhcl.Wheel.RL/1(Out1) -> Vhcl.Wheel.RL/1  "Vhcl.Wheel.RL"
  CreateBus Vhcl.Wheel.RR/1(Out1) -> Vhcl.Wheel.RR/1  "Vhcl.Wheel.RR"
  Trailer/8 -> CreateBus Vhcl.Wheel.RR/1(In1)
  Trailer/7 -> CreateBus Vhcl.Wheel.RL/1(In1)
  Trailer/6 -> CreateBus Vhcl.Wheel.FR/1(In1)
  Trailer/5 -> CreateBus Vhcl.Wheel.FL/1(In1)
  Trailer/17 -> CreateBus Car.Hitch.FrcTrq/1(In1)
  Trailer/2 -> CreateBus Vhcl.Steering/1(In1)
  CreateBus Vhcl.Steering/1(Out1) -> Vhcl.Steering/1  "Vhcl.Steering"
  Trailer/3 -> CreateBus Vhcl.Motion/1(In1)
  Trailer/4 -> CreateBus Vhcl.PoI/1(In1)
  CreateBus Vhcl.PoI/1(Out1) -> Vhcl.PoI/1  "Vhcl.PoI"
  CreateBus Vhcl.Motion/1(Out1) -> Vhcl.Motion/1  "Vhcl.Motion"
  Car.Trq_T2W/1 -> Trailer/5
  WheelCarrier.Misc/1 -> Trailer/6
  CreateBus Car.Hitch.FrcTrq/1(Out1) -> Car.Hitch.FrcTrq/1  "Car.Hitch.FrcTrq"
  Car.Fr1/1 -> Trailer/4
  Car.Hitch/1 -> Trailer/3
  Trailer.Load/1 -> Trailer/2
  Trailer/1 -> Sync_Out/1
  Sync_In/1 -> Trailer/1

== system generic_Truck_And_Trailer/TruckMaker/Subsystem1/ONE_TRACK_MODEL_TRACTOR_UKF/Measurements from IMU ==
  Acc_x : TruckMaker4SL/Read CM Dict  xname=Sensor.Inertial.Vhcl.VchBdy.Acc_B.x  xsync=off  xstime=Continuous
      settings: SourceProductName=TruckMaker4SL
  Acc_y : TruckMaker4SL/Read CM Dict  xname=Sensor.Inertial.Vhcl.VchBdy.Acc_B.y  xsync=off  xstime=Continuous
      settings: SourceProductName=TruckMaker4SL
  Omega_z : TruckMaker4SL/Read CM Dict  xname=Sensor.Inertial.Vhcl.VchBdy.Omega_B.z  xsync=off  xstime=Continuous
      settings: SourceProductName=TruckMaker4SL
  Vel_x : TruckMaker4SL/Read CM Dict  xname=Sensor.Inertial.Vhcl.VchBdy.Vel_B.x  xsync=off  xstime=Continuous
      settings: SourceProductName=TruckMaker4SL
  Vel_y : TruckMaker4SL/Read CM Dict  xname=Sensor.Inertial.Vhcl.VchBdy.Vel_B.y  xsync=off  xstime=Continuous
      settings: SourceProductName=TruckMaker4SL
  acc_x : Outport
  acc_y : Outport  Port=2
  vel_x : Outport  Port=3
  vel_y : Outport  Port=4
  wz : Outport  Port=5
  wires:
  Omega_z/1 -> wz/1
  Vel_x/1 -> vel_x/1
  Vel_y/1 -> vel_y/1
  Acc_x/1 -> acc_x/1
  Acc_y/1 -> acc_y/1

== system generic_Truck_And_Trailer/TruckMaker/Subsystem1/Subsystem/Ackerman Angle ==
  MATLAB Function : MATLAB Function  TreatAsAtomicUnit=on
  Read CM Dict11 : TruckMaker4SL/Read CM Dict  xname=Car.SteerAngleFR  xsync=off  xstime=Continuous
      settings: SourceProductName=TruckMaker4SL
  Read CM Dict6 : TruckMaker4SL/Read CM Dict  xname=Car.SteerAngleFL  xsync=off  xstime=Continuous
      settings: SourceProductName=TruckMaker4SL
  Out1 : Outport
  wires:
  Read CM Dict11/1 -> MATLAB Function/2(delta_r)
  Read CM Dict6/1 -> MATLAB Function/1(delta_l)
  MATLAB Function/1(delta) -> Out1/1

== system generic_Truck_And_Trailer/TruckMaker/Subsystem1/Subsystem/Average Steering Angle ==
  Gain : Gain  Gain=0.5
  Read CM Dict11 : TruckMaker4SL/Read CM Dict  xname=Car.SteerAngleFR  xsync=off  xstime=Continuous
      settings: SourceProductName=TruckMaker4SL
  Read CM Dict6 : TruckMaker4SL/Read CM Dict  xname=Car.SteerAngleFL  xsync=off  xstime=Continuous
      settings: SourceProductName=TruckMaker4SL
  Sum : Sum  Inputs=|++
  "Average_steering " : Outport
  wires:
  Read CM Dict6/1 -> Sum/2
  Sum/1 -> Gain/1
  Read CM Dict11/1 -> Sum/1
  Gain/1 -> "Average_steering "/1

== system generic_Truck_And_Trailer/TruckMaker/Subsystem1/Subsystem/Bromsmoment  trailer rear ==
  FYh1 : TruckMaker4SL/Read CM Dict  xname=Tr.Brake.Trq_WB_FL  xsync=off  xstime=Continuous
      settings: SourceProductName=TruckMaker4SL
  FYh2 : TruckMaker4SL/Read CM Dict  xname=Tr.Brake.Trq_WB_FR  xsync=off  xstime=Continuous
      settings: SourceProductName=TruckMaker4SL
  Gain : Gain
  Sum : Sum  Inputs=|++
  "Average_Bromsmomet " : Outport
  wires:
  Gain/1 -> "Average_Bromsmomet "/1
  FYh1/1 -> Sum/1
  Sum/1 -> Gain/1
  FYh2/1 -> Sum/2

== system generic_Truck_And_Trailer/TruckMaker/Subsystem1/Subsystem/Bromsmoment fram  ==
  FYh1 : TruckMaker4SL/Read CM Dict  xname=Brake.Trq_WB_FL  xsync=off  xstime=Continuous
      settings: SourceProductName=TruckMaker4SL
  FYh2 : TruckMaker4SL/Read CM Dict  xname=Brake.Trq_WB_FR  xsync=off  xstime=Continuous
      settings: SourceProductName=TruckMaker4SL
  Sum : Sum  Inputs=|++
  "Average_Bromsmomet " : Outport
  wires:
  Sum/1 -> "Average_Bromsmomet "/1
  FYh1/1 -> Sum/1
  FYh2/1 -> Sum/2

== system generic_Truck_And_Trailer/TruckMaker/Subsystem1/Subsystem/Bromsmoment rear 1 ==
  FYh1 : TruckMaker4SL/Read CM Dict  xname=Brake.Trq_WB_RL  xsync=off  xstime=Continuous
      settings: SourceProductName=TruckMaker4SL
  FYh2 : TruckMaker4SL/Read CM Dict  xname=Brake.Trq_WB_RR  xsync=off  xstime=Continuous
      settings: SourceProductName=TruckMaker4SL
  Sum : Sum  Inputs=|++
  "Average_Bromsmomet " : Outport
  wires:
  FYh2/1 -> Sum/2
  FYh1/1 -> Sum/1
  Sum/1 -> "Average_Bromsmomet "/1

== system generic_Truck_And_Trailer/TruckMaker/Subsystem1/Subsystem_Noisey Measurements/Measurements from IMU ==
  Acc_x : TruckMaker4SL/Read CM Dict  xname=Sensor.Inertial.Vhcl.VchBdy.Acc_B.x  xsync=off  xstime=Continuous
      settings: SourceProductName=TruckMaker4SL
  Acc_y : TruckMaker4SL/Read CM Dict  xname=Sensor.Inertial.Vhcl.VchBdy.Acc_B.y  xsync=off  xstime=Continuous
      settings: SourceProductName=TruckMaker4SL
  Acc_z : TruckMaker4SL/Read CM Dict  xname=Sensor.Inertial.Vhcl.VchBdy.Acc_B.z  xsync=off  xstime=Continuous
      settings: SourceProductName=TruckMaker4SL
  Omega_z : TruckMaker4SL/Read CM Dict  xname=Sensor.Inertial.Vhcl.VchBdy.Omega_B.z  xsync=off  xstime=Continuous
      settings: SourceProductName=TruckMaker4SL
  Omega_z1 : TruckMaker4SL/Read CM Dict  xname=Sensor.Inertial.Vhcl.VchBdy.Omega_B.y  xsync=off  xstime=Continuous
      settings: SourceProductName=TruckMaker4SL
  Omega_z2 : TruckMaker4SL/Read CM Dict  xname=Sensor.Inertial.Vhcl.VchBdy.Omega_B.x  xsync=off  xstime=Continuous
      settings: SourceProductName=TruckMaker4SL
  Vel_x : TruckMaker4SL/Read CM Dict  xname=Sensor.Inertial.Vhcl.VchBdy.Vel_B.x  xsync=off  xstime=Continuous
      settings: SourceProductName=TruckMaker4SL
  Vel_y : TruckMaker4SL/Read CM Dict  xname=Sensor.Inertial.Vhcl.VchBdy.Vel_B.y  xsync=off  xstime=Continuous
      settings: SourceProductName=TruckMaker4SL
  Vel_z : TruckMaker4SL/Read CM Dict  xname=Sensor.Inertial.Vhcl.VchBdy.Vel_B.z  xsync=off  xstime=Continuous
      settings: SourceProductName=TruckMaker4SL
  acc_x : Outport
  acc_y : Outport  Port=2
  acc_z : Outport  Port=3
  vel_x : Outport  Port=4
  vel_y : Outport  Port=5
  vel_z : Outport  Port=6
  wx : Outport  Port=7
  wy : Outport  Port=8
  wz : Outport  Port=9
  wires:
  Acc_x/1 -> acc_x/1
  Acc_y/1 -> acc_y/1
  Acc_z/1 -> acc_z/1
  Vel_x/1 -> vel_x/1
  Vel_y/1 -> vel_y/1
  Vel_z/1 -> vel_z/1
  Omega_z2/1 -> wx/1
  Omega_z1/1 -> wy/1
  Omega_z/1 -> wz/1

== system generic_Truck_And_Trailer/TruckMaker/Subsystem1/Subsystem_Noisey Measurements _NAN/Measurements from IMU ==
  Acc_x : TruckMaker4SL/Read CM Dict  xname=Sensor.Inertial.Vhcl.VchBdy.Acc_B.x  xsync=off  xstime=Continuous
      settings: SourceProductName=TruckMaker4SL
  Acc_y : TruckMaker4SL/Read CM Dict  xname=Sensor.Inertial.Vhcl.VchBdy.Acc_B.y  xsync=off  xstime=Continuous
      settings: SourceProductName=TruckMaker4SL
  Acc_z : TruckMaker4SL/Read CM Dict  xname=Sensor.Inertial.Vhcl.VchBdy.Acc_B.z  xsync=off  xstime=Continuous
      settings: SourceProductName=TruckMaker4SL
  Omega_z : TruckMaker4SL/Read CM Dict  xname=Sensor.Inertial.Vhcl.VchBdy.Omega_B.z  xsync=off  xstime=Continuous
      settings: SourceProductName=TruckMaker4SL
  Omega_z1 : TruckMaker4SL/Read CM Dict  xname=Sensor.Inertial.Vhcl.VchBdy.Omega_B.y  xsync=off  xstime=Continuous
      settings: SourceProductName=TruckMaker4SL
  Omega_z2 : TruckMaker4SL/Read CM Dict  xname=Sensor.Inertial.Vhcl.VchBdy.Omega_B.x  xsync=off  xstime=Continuous
      settings: SourceProductName=TruckMaker4SL
  Vel_x : TruckMaker4SL/Read CM Dict  xname=Sensor.Inertial.Vhcl.VchBdy.Vel_B.x  xsync=off  xstime=Continuous
      settings: SourceProductName=TruckMaker4SL
  Vel_y : TruckMaker4SL/Read CM Dict  xname=Sensor.Inertial.Vhcl.VchBdy.Vel_B.y  xsync=off  xstime=Continuous
      settings: SourceProductName=TruckMaker4SL
  Vel_z : TruckMaker4SL/Read CM Dict  xname=Sensor.Inertial.Vhcl.VchBdy.Vel_B.z  xsync=off  xstime=Continuous
      settings: SourceProductName=TruckMaker4SL
  acc_x : Outport
  acc_y : Outport  Port=2
  acc_z : Outport  Port=3
  vel_x : Outport  Port=4
  vel_y : Outport  Port=5
  vel_z : Outport  Port=6
  wx : Outport  Port=7
  wy : Outport  Port=8
  wz : Outport  Port=9
  wires:
  Omega_z/1 -> wz/1
  Omega_z1/1 -> wy/1
  Omega_z2/1 -> wx/1
  Vel_z/1 -> vel_z/1
  Vel_y/1 -> vel_y/1
  Vel_x/1 -> vel_x/1
  Acc_z/1 -> acc_z/1
  Acc_y/1 -> acc_y/1
  Acc_x/1 -> acc_x/1

== system generic_Truck_And_Trailer/TruckMaker/Tractor_Subsystem /ONE_TRACK_MODEL_TRACTOR_UKF/Measurements from IMU ==
  Acc_x : TruckMaker4SL/Read CM Dict  xname=Sensor.Inertial.Vhcl.VchBdy.Acc_B.x  xsync=off  xstime=Continuous
      settings: SourceProductName=TruckMaker4SL
  Acc_y : TruckMaker4SL/Read CM Dict  xname=Sensor.Inertial.Vhcl.VchBdy.Acc_B.y  xsync=off  xstime=Continuous
      settings: SourceProductName=TruckMaker4SL
  Omega_z : TruckMaker4SL/Read CM Dict  xname=Sensor.Inertial.Vhcl.VchBdy.Omega_B.z  xsync=off  xstime=Continuous
      settings: SourceProductName=TruckMaker4SL
  Vel_x : TruckMaker4SL/Read CM Dict  xname=Sensor.Inertial.Vhcl.VchBdy.Vel_B.x  xsync=off  xstime=Continuous
      settings: SourceProductName=TruckMaker4SL
  Vel_y : TruckMaker4SL/Read CM Dict  xname=Sensor.Inertial.Vhcl.VchBdy.Vel_B.y  xsync=off  xstime=Continuous
      settings: SourceProductName=TruckMaker4SL
  acc_x : Outport
  acc_y : Outport  Port=2
  vel_x : Outport  Port=3
  vel_y : Outport  Port=4
  wz : Outport  Port=5
  wires:
  Acc_y/1 -> acc_y/1
  Acc_x/1 -> acc_x/1
  Vel_y/1 -> vel_y/1
  Vel_x/1 -> vel_x/1
  Omega_z/1 -> wz/1

== system generic_Truck_And_Trailer/TruckMaker/Tractor_Subsystem /Subsystem/Ackerman Angle ==
  MATLAB Function : MATLAB Function  TreatAsAtomicUnit=on
  Read CM Dict11 : TruckMaker4SL/Read CM Dict  xname=Car.SteerAngleFR  xsync=off  xstime=Continuous
      settings: SourceProductName=TruckMaker4SL
  Read CM Dict6 : TruckMaker4SL/Read CM Dict  xname=Car.SteerAngleFL  xsync=off  xstime=Continuous
      settings: SourceProductName=TruckMaker4SL
  Out1 : Outport
  wires:
  MATLAB Function/1(delta) -> Out1/1
  Read CM Dict6/1 -> MATLAB Function/1(delta_l)
  Read CM Dict11/1 -> MATLAB Function/2(delta_r)

== system generic_Truck_And_Trailer/TruckMaker/Tractor_Subsystem /Subsystem/Average Steering Angle ==
  Gain : Gain  Gain=0.5
  Read CM Dict11 : TruckMaker4SL/Read CM Dict  xname=Car.SteerAngleFR  xsync=off  xstime=Continuous
      settings: SourceProductName=TruckMaker4SL
  Read CM Dict6 : TruckMaker4SL/Read CM Dict  xname=Car.SteerAngleFL  xsync=off  xstime=Continuous
      settings: SourceProductName=TruckMaker4SL
  Sum : Sum  Inputs=|++
  "Average_steering " : Outport
  wires:
  Gain/1 -> "Average_steering "/1
  Read CM Dict11/1 -> Sum/1
  Sum/1 -> Gain/1
  Read CM Dict6/1 -> Sum/2
